simulink model "model_izhikevich"  (R2020b)
settings: Solver=VariableStepAuto  StartTime=15  StopTime=10  RelTol=1e-3
settings Model: Creator=a1  LastModifiedBy=a1
settings HardwareCC: ProdBitPerLong=64  ProdHWDeviceType=Intel->x86-64 (Mac OS X)

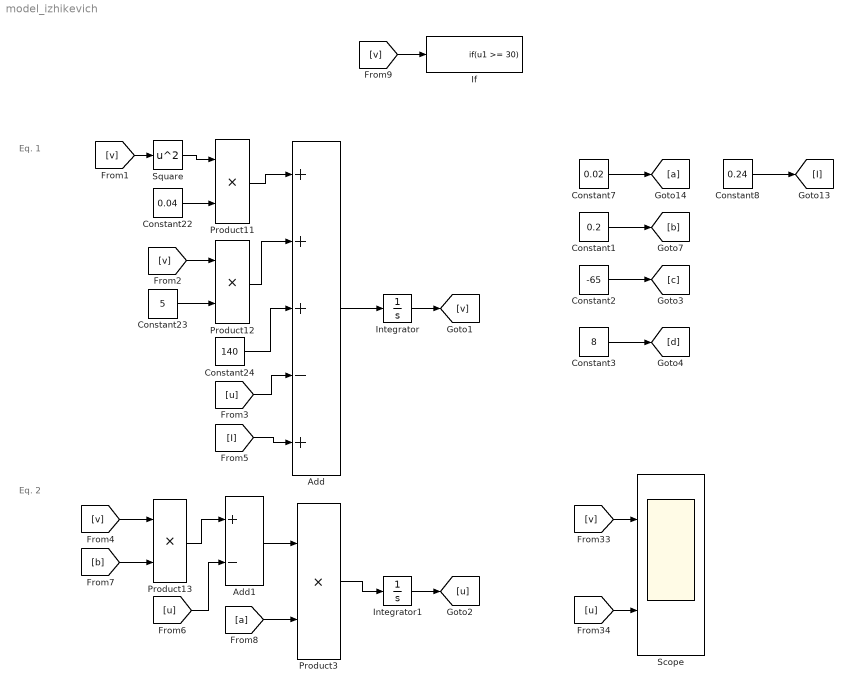
== system model_izhikevich ==
  note: Eq. 1
  note: Eq. 2
  Add : Sum  Inputs=+++-+
  Add1 : Sum  Inputs=+-
  Constant1 : Constant  Value=0.2
  Constant2 : Constant  Value=-65
  Constant22 : Constant  Value=0.04
  Constant23 : Constant  Value=5
  Constant24 : Constant  Value=140
  Constant3 : Constant  Value=8
  Constant7 : Constant  Value=0.02
  Constant8 : Constant  Value=0.24
  If : If  IfExpression=u1 >= 30  ShowElse=off
  Integrator : Integrator
  Integrator1 : Integrator
  Product11 : Product
  Product12 : Product
  Product13 : Product
  Product3 : Product  Inputs=**
  Scope : Scope  NumInputPorts=2
  Square : Math  Operator=square  SaturateOnIntegerOverflow=on
  wires:
  Integrator/1 -> [v]
  Add1/1 -> Product3/1
  [u] -> Add1/2
  Product3/1 -> Integrator1/1
  Integrator1/1 -> [u]
  Constant1/1 -> [b]
  Constant8/1 -> [I]
  Constant7/1 -> [a]
  [v] -> Scope/1
  [u] -> Scope/2
  [v] -> Square/1
  Square/1 -> Product11/1
  Constant22/1 -> Product11/2
  Product11/1 -> Add/1
  Constant23/1 -> Product12/2
  [v] -> Product12/1
  Product12/1 -> Add/2
  Constant24/1 -> Add/3
  [u] -> Add/4
  Add/1 -> Integrator/1
  [v] -> Product13/1
  Product13/1 -> Add1/1
  [I] -> Add/5
  [b] -> Product13/2
  [a] -> Product3/2
  Constant2/1 -> [c]
  Constant3/1 -> [d]
  [v] -> If/1
